simulink library "resettableCounter"  (R2018a)
settings: Solver=VariableStepAuto  StartTime=0.0  StopTime=10.0  RelTol=1e-3
libraries: simulink x1
settings Model: Creator=mitch  LastModifiedBy=mitch

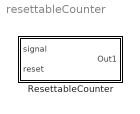
== system resettableCounter ==
  ResettableCounter : Subsystem

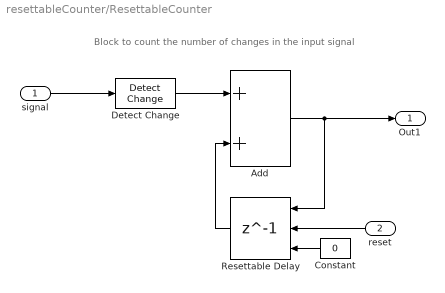
== system resettableCounter/ResettableCounter ==
  note: Block to count the number of changes in the input signal
  signal : Inport
  reset : Inport  Port=2
  Add : Sum
  Constant : Constant  Value=0
  Detect Change : simulink/Logic and Bit Operations/Detect Change  vinit=0  OutDataTypeStr=boolean
  Resettable Delay : Delay  DelayLength=1  InitialConditionSource=Input port  ExternalReset=Rising
      settings: InputPortMap=u0,r5,p4
  Out1 : Outport
  wires:
  Add/1 -> Resettable Delay/1, Out1/1
  Resettable Delay/1 -> Add/2
  reset/1 -> Resettable Delay/2
  Constant/1 -> Resettable Delay/3
  Detect Change/1 -> Add/1
  signal/1 -> Detect Change/1
